simulink library "AeroLib"  (Simulink 6.0)
settings: Solver=ode45  SolverMode=SingleTasking  StartTime=0.0  StopTime=10.0  RelTol=1e-3
undefined symbols (not defined in the file): Aero, Ap, Atm, Control, Controls, Eng, Flight_cg, Flight_DamperON, Flight_delta_isa, Flight_DeltaSpiral, Flight_InertiaSelect, Flight_ixx, Flight_ixz, Flight_iyy, Flight_izz, Flight_latitude, Flight_LoiterLenght, Flight_LoiterMode, Flight_LoiterRadius, Flight_longitude, Flight_MaxTargetPoints, Flight_SensorsON, Flight_TimeStep, Flight_TowerWind_X, Flight_TowerWind_Y, Flight_TowerWind_Z, Flight_TowerWindON, Flight_Trimming, Flight_TurbON, Flight_weight, Flight_WindGustON, Flight_WindShearON, Flight_ycg, Flight_zcg, Geom, Lgear, Mass, PEG_CDwbnp, PEG_CLht, PEG_CLht_elev, PEG_CLwbnp, PEG_CMht, PEG_CMwbnp, PEG_CNbeta, PEG_CNr, PEG_CNrud, PEG_CRail, PEG_CRbeta, PEG_CRp, PEG_CRrud, PEG_CYbeta, PEG_CYrud, pow, Sensors
libraries: AeroLib x133, simulink3 x49, simulink x37, aerospace x11
(part 1 of 7)
settings Model: LastModifiedBy=MarcoP
settings OptimizationCC: BooleanDataType=off
settings DebuggingCC: SolverPrmCheckMsg=none
settings HardwareCC: TargetUnknown=on

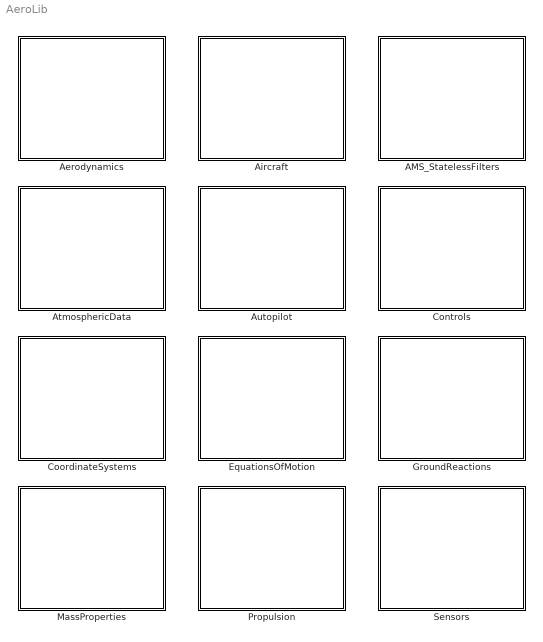
== system AeroLib ==
  AMS_StatelessFilters : Subsystem
      mask Display: image(imread('Filters.bmp','bmp'))
  Aerodynamics : Subsystem
      mask Display: image(imread('Aero.bmp','bmp'))
  Aircraft : Subsystem
      mask Type: Aircraft library
      mask Display: image(imread('Aircraft.bmp','bmp'))
  AtmosphericData : Subsystem
      mask Display: image(imread('Atm.bmp','bmp'))
  Autopilot : Subsystem
      mask Display: image(imread('Autopilot.bmp','bmp'))
  Controls : Subsystem
      mask Display: image(imread('Ctrl.bmp','bmp'))
  CoordinateSystems : Subsystem
      mask Display: image(imread('CoordSys.bmp','bmp'))
  EquationsOfMotion : Subsystem
      mask Display: image(imread('EQM.bmp','bmp'))
  GroundReactions : Subsystem
      mask Display: image(imread('Ground.bmp','bmp'))
  MassProperties : Subsystem
      mask Display: image(imread('Mass.bmp','bmp'))
  Propulsion : Subsystem
      mask Display: image(imread('Prop.bmp','bmp'))
  Sensors : Subsystem
      mask Display: image(imread('Sensors.bmp','bmp'))

== system AeroLib/AMS_StatelessFilters ==
  note: NB: The high pass has a
      | gain error of tau at high frequencies
  FlightTrim_Switch : Subsystem
      mask Help: See AeroLib Reference Manual.
      mask Display: patch([0 0.45 0.45 0.55 0.55 1], [0 0 1 1 0 0], [0 0 0]);
  Stateless_Filter_Reset : Subsystem
      mask Help: See AeroLib Reference Manual.
      mask Display: patch([0 0.45 0.45 0.55 0.55 1], [0 0 1 1 0 0], [0 0 0]);
  Stateless_HighPass : Subsystem
      mask Help: See AeroLib Reference Manual.
      mask Display: patch([0 0.4 0.4 0.6 0.6 1], [0 0 1 1 0 0], [0 0 0]);
  Stateless_Integrator : Subsystem
      mask Help: See AeroLib Reference Manual.
      mask Display: patch([0 0.4 0.4 0.6 0.6 1], [0 0 1 1 0 0], [0 0 0]);
  Stateless_LeadLag : Subsystem
      mask Help: See AeroLib Reference Manual.
      mask Display: patch([0 0.4 0.4 0.6 0.6 1], [0 0 1 1 0 0], [0 0 0]);
  Stateless_LimIntegrator : Subsystem
      mask Help: See AeroLib Reference Manual.
      mask Display: patch([0 0.4 0.4 0.6 0.6 1], [0 0 1 1 0 0], [0 0 0]);
  Stateless_LowPass : Subsystem
      mask Help: See AeroLib Reference Manual.
      mask Display: patch([0 0.4 0.4 0.6 0.6 1], [0 0 1 1 0 0], [0 0 0]);
  Stateless_RateLimiter : Subsystem
      mask Help: See AeroLib Reference Manual.
      mask Display: patch([0 0.4 0.4 0.6 0.6 1], [0 0 1 1 0 0], [0 0 0]);

== system AeroLib/Aerodynamics ==
  Aero NonDim_Rates : Subsystem  mask{Bref=Geom.Wing.bref, Cref=Geom.Wing.cref}
      mask prompts: Bref "Wing Span"; Cref "Wing MAC"
  Aerodynamic_Linear_Static : Subsystem
  Aerodynamics_Generic : Subsystem
      mask Help: See AeroLib Reference Manual.
      mask Display: patch( [0 0.4 0.4 0.6 0.6 1], [0 0 1 1 0 0],  [1 0 0])
  Aerodynamics_Pioneer : Subsystem
      mask Help: See AeroLib Reference Manual.
      mask Display: patch( [0 0.4 0.4 0.6 0.6 1], [0 0 1 1 0 0],  [1 0 0])
  INIT_Arms : Subsystem  mask{zacnp=Geom.Nacelle.zacnp, xacnp=Geom.Nacelle.xacnp, zacvt=Geom.Vtail.zacvt, xacvt=Geom.Vtail.xacvt, zacht=Geom.Htail.zacht, yacht=Geom.Htail.yacht, xacht=Geom.Htail.xacht, Cref=Geom.Wing.cref, Bref=Geom.Wing.bref}
      mask prompts: zacnp "(znp - zac)/span"; xacnp "(xnp - xac)/span"; zacvt "(zacvt -zac)/span"; xacvt "(xacvt - xac)/span"; zacht "(zacht -zac)/mac"; yacht "(yacht -yac)/span"; xacht "(xacht - xac)/mac"; Cref "Wing MAC"; Bref "Wing Span"
      mask help:
      | Htail - Horizontal Tail
      | Vtail - Vertical Tail
      | np - nacelle pilon
  Loads : Subsystem  mask{Bref=Geom.Wing.bref, Cref=Geom.Wing.cref, Sw=Geom.Wing.sw}
      mask prompts: Bref "Wing Span"; Cref "Wing MAC"; Sw "Wing Area"
  Transf to CG : Subsystem  mask{Bref=Geom.Wing.bref, Cref=Geom.Wing.cref}
      mask prompts: Bref "Wing Span"; Cref "Wing MAC"

== system AeroLib/Aircraft ==
  Generic_Aircraft : Subsystem
      mask Help: See AeroLib Reference Manual.
      mask Display:
      | patch( [0 0.07 0.19 0.09 0.02 0.07 0], [1 0.6 0.6 0.75 0.75 0.6 1], [0 0.7 1])
      | patch( [0 0.09 0.21 0.07 0], [0.52 0.52 0.6 0.6 0.52], [0 0.7 1])
      | patch( [0 0.25 0.37 0.59 0.4 0.25 0], [0 0.32 0.32 0.5 0.5 0.32 0], [0 0.7 1])
      | patch( [0.21 0.86 0.86 0.07 0.21], [0.5 0.5 0.6 0.6 0.5], [0 0.7 1])
      | patch( [0.86 1 1 0.86 0.86], [0.5 0.5 0.52 0.6 0.5], [0 0.7 1])
      | patch( [0.48 0.67 0.75 0.65 0.48], [0.6 0.6 0.7 0.7 0.6], [0 0.7 1])
  Pioneer_Aircraft : Subsystem
      mask Help: See AeroLib Reference Manual.
      mask Display:
      | patch( [0 0.07 0.19 0.09 0.02 0.07 0], [1 0.6 0.6 0.75 0.75 0.6 1], [0 0.7 1])
      | patch( [0 0.09 0.21 0.07 0], [0.52 0.52 0.6 0.6 0.52], [0 0.7 1])
      | patch( [0 0.25 0.37 0.59 0.4 0.25 0], [0 0.32 0.32 0.5 0.5 0.32 0], [0 0.7 1])
      | patch( [0.21 0.86 0.86 0.07 0.21], [0.5 0.5 0.6 0.6 0.5], [0 0.7 1])
      | patch( [0.86 1 1 0.86 0.86], [0.5 0.5 0.52 0.6 0.5], [0 0.7 1])
      | patch( [0.48 0.67 0.75 0.65 0.48], [0.6 0.6 0.7 0.7 0.6], [0 0.7 1])

== system AeroLib/AtmosphericData ==
  Atmosphere : Subsystem  mask{ISA=Flight_delta_isa, g=9.806, gamma=1.4, R=287.0529, L=0.0065, h_trop=11000, P0=101325.0, T0=288.15}
      mask prompts: ISA "Delta_ISA_C"; g "Gravity Acceleration [m/s2]"; gamma "Ratio of Specific Heats"; R "Characteristic Gas Constant [J/Kg/K]"; L "Lapse Rate [K/m]"; h_trop "Height of Troposphere [m]"; P0 "Pressure at sea level [N/m2]"; T0 "Ambient Temperature at Sea Level [K]"
      mask Display: patch([0 0.45 0.45 0.55 0.55 1], [0 0 1 1 0 0], [0 0.9 0.2])
  AtmosphericData_FAA_gust : Subsystem
      settings: RTWSystemCode=Function  RTWFcnNameOpts=Use subsystem name  RTWFileNameOpts=Use subsystem name
      mask Help: See AeroLib Reference Manual.
      mask Display: patch( [0 0.4 0.4 0.6 0.6 1], [0 0 1 1 0 0],  [0 0.9 0.2])
  FAA_Std_Gust : Subsystem
      mask Help: See AeroLib Reference Manual.
      mask Display: patch(  [0 0.45 0.45 0.55 0.55 1], [0 0 1 1 0 0],  [0 0.9 0.2])
  Simple_Wind_Gust : Subsystem  mask{WGfac=3, F=2.5, Wgain=-0.05}
      mask Help: See AeroLib Reference Manual.
      mask Display: patch(  [0 0.45 0.45 0.55 0.55 1], [0 0 1 1 0 0],  [0 0.9 0.2])

== system AeroLib/Autopilot ==
  AutoPilot_Out : Subsystem
      mask Display: disp('Empty')
  Autopilot : Subsystem
      settings: RTWSystemCode=Function  RTWFcnNameOpts=Use subsystem name  RTWFileNameOpts=Use subsystem name
      mask Help: See AeroLib Reference Manual.
      mask Display: patch( [0 0.4 0.4 0.6 0.6 1], [0 0 1 1 0 0],  [0 0.7 1])
  Counter_Point : Subsystem  mask{MinDist=Ap.Target.MinDist}
      mask prompts: MinDist "Minimal Distance"
  GeodCoor to XY : Subsystem
  Geod_Target_Errors : Subsystem
  PID : Subsystem  mask(PID(2) Controller){P=Ap.Alt.pgain, I=Ap.Alt.igain, D=0, Lim_I=Ap.Alt.igainLim, Lim_Err=Ap.Alt.LimAlt, Lim_Com=50}
      mask prompts: P "Proportional:"; I "Integral:"; D "Derivative:"; Lim_I "Limit Integral"; Lim_Err "Limit Error"; Lim_Com "Limit Comand"
      mask help:
      | Enter Proportional(P), Integral(I), and Derivative(D) terms.
      | P+I/s+Ds
      mask Help: This block implements a PID controller where parameters are entered for the Proportional, Integral and Derivative and divisor terms. Unmask this block to see how it works. The derivative term is implemented using an s/(s/N +1)  transfer function block. Making N large can create a "stiff" system.
      mask Display: disp('PID')
  Target_Errors : Subsystem

== system AeroLib/Controls ==
  Simple_Aileron_Actuator : Subsystem  mask{tau=Controls.Ail.Gain, ratio=Control.Wheel.Ratio, up=Controls.Ail.MaxAngle, low=-Controls.Ail.MaxAngle}
      mask prompts: tau "Time constant"; ratio "Aileron ratio"; up "Up limit"; low "Low limit"
      mask Help: See AeroLib Reference Manual.
      mask Display: patch( [0 0.5 0.5 0 0 0.5 0.5 1 0 0], [0 0 0.2 0.2 0.8 0.8 1 1 1 0],  [1 1 0.6])
  Simple_Controls : Subsystem
      mask Help: See AeroLib Reference Manual.
      mask Display: patch( [0 0.4 0.4 0.6 0.6 1], [0 0 1 1 0 0], [1 0 0.8])
  Simple_Elevator_Actuator : Subsystem  mask{tau=Controls.Elev.Gain, up=Controls.Elev.MaxPos, low=Controls.Elev.MaxNeg}
      mask prompts: tau "Time constant"; up "Up limit"; low "Low limit"
      mask Help: See AeroLib Reference Manual.
      mask Display: patch( [0 0.5 0.5 0 0 0.5 0.5 1 0 0], [0 0 0.2 0.2 0.8 0.8 1 1 1 0],  [1 1 0.6])
  Simple_Flap_Actuator : Subsystem  mask{flap_pos=Controls.flapslat, flap_defl=Controls.flap.Defl, flap_rate=Controls.flap.Rate}
      mask prompts: flap_pos "Flap Position"; flap_defl "Flap Deflection"; flap_rate "Flap Rate Limit"
      mask Help: See AeroLib Reference Manual.
      mask Display: patch( [0 0.5 0.5 0 0 0.5 0.5 1 0 0], [0 0 0.1 0.1 0.9 0.9 1 1 1 0],  [1 1 0.6])
  Simple_Rudder_Actuator : Subsystem  mask{tau=Controls.Rudder.Gain, up=Controls.Rudder.MaxAngle, low=-Controls.Rudder.MaxAngle}
      mask prompts: tau "Time constant"; up "Up limit"; low "Low limit"
      mask Help: See AeroLib Reference Manual.
      mask Display: patch( [0 0.5 0.5 0 0 0.5 0.5 1 0 0], [0 0 0.2 0.2 0.8 0.8 1 1 1 0],  [1 1 0.6])
  Simple_Stab_Actuator : Subsystem  mask{gain=Controls.Stab.Gain, up=Controls.Stab.MaxPos, low=Controls.Stab.MaxNeg}
      mask prompts: up "Up Limit"; low "Low Limit"
      mask Help: See AeroLib Reference Manual.
      mask Display: patch( [0 0.5 0.5 0 0 0.5 0.5 1 0 0], [0 0 0.2 0.2 0.8 0.8 1 1 1 0],  [1 1 0.6])

== system AeroLib/CoordinateSystems ==
  BOA2LEF : Subsystem
      settings: RTWSystemCode=Function  RTWFcnNameOpts=Use subsystem name  RTWFileNameOpts=Use subsystem name
      mask Help: See AeroLib Reference Manual.
      mask Display: patch( [0 0.5 0.5 1 1 0.5 0.5 1 1 0.5], [0 0 1 1 0.6 0.6 0.4 0.4 0 0], [1 1 0.6])
  EUL2DCM : Subsystem
      settings: RTWSystemCode=Function  RTWFcnNameOpts=Use subsystem name  RTWFileNameOpts=Use subsystem name
      mask Help: See AeroLib Reference Manual.
      mask Display: patch( [0 0.5 0.5 0 0 0.5 0.5 1 0 0], [0 0 0.4 0.4 0.6 0.6 1 1 1 0], [1 0 0])
  EUL2QUA : Subsystem
      settings: RTWSystemCode=Function  RTWFcnNameOpts=Use subsystem name  RTWFileNameOpts=Use subsystem name
      mask Help: See AeroLib Reference Manual.
      mask Display: patch( [0 0.5 0.5 0 0 0.5 0.5 1 0 0], [0 0 0.4 0.4 0.6 0.6 1 1 1 0], [0 0 .9])
  QUA2DCM : Subsystem
      settings: RTWSystemCode=Function  RTWFcnNameOpts=Use subsystem name  RTWFileNameOpts=Use subsystem name
      mask Help: See AeroLib Reference Manual.
      mask Display: patch( [0 0.5 0.5 1 1 0.5 0.5 1 1 0.5], [0 0 1 1 0.6 0.6 0.4 0.4 0 0], [1 0 0])
  QUA2EUL : Subsystem
      settings: RTWSystemCode=Function  RTWFcnNameOpts=Use subsystem name  RTWFileNameOpts=Use subsystem name
      mask Help: See AeroLib Reference Manual.
      mask Display: patch( [0 0.5 0.5 1 1 0.5 0.5 1 1 0.5], [0 0 1 1 0.6 0.6 0.4 0.4 0 0], [0 0 .9])
  STA2BOA : Subsystem
      settings: RTWSystemCode=Function  RTWFcnNameOpts=Use subsystem name  RTWFileNameOpts=Use subsystem name
      mask Help: See AeroLib Reference Manual.
      mask Display: patch( [0 0.5 0.5 1 1 0.5 0.5 1 1 0.5], [0 0 1 1 0.6 0.6 0.4 0.4 0 0], [1 1 0.6])
  WND2STA : Subsystem
      settings: RTWSystemCode=Function  RTWFcnNameOpts=Use subsystem name  RTWFileNameOpts=Use subsystem name
      mask Help: See AeroLib Reference Manual.
      mask Display: patch( [0 0.5 0.5 1 1 0.5 0.5 1 1 0.5], [0 0 1 1 0.6 0.6 0.4 0.4 0 0], [1 1 0.6])

== system AeroLib/EquationsOfMotion ==
  Equations_of_Motion : Subsystem
      mask Type: SampleMaskedBlock
      mask Help: See AeroLib Reference Manual.
      mask Display: patch( [0 0.5 0.5 1 1 0.5 0.5 1 1 0.5], [0 0 1 1 0.6 0.6 0.4 0.4 0 0], [0 0 1])
  External_Forces_and_Moments : Subsystem
      mask Help: See AeroLib Reference Manual.
      mask Display: patch( [0 0.5 0.5 1 1 0.5 0.5 1 1 0.5], [0 0 1 1 0.92 0.92 0.08 0.08 0 0], [0 0 1])

== system AeroLib/GroundReactions ==
  Gear_Out : Subsystem
      mask Display: disp('Empty')
  Landing_Gear : Subsystem
      settings: RTWSystemCode=Function  RTWFcnNameOpts=Use subsystem name  RTWFileNameOpts=Use subsystem name
      mask Help: See AeroLib Reference Manual.
      mask Display: patch( [0 0.4 0.4 0.6 0.6 1], [0 0 1 1 0 0],  [.8 0.8 .8])

== system AeroLib/MassProperties ==
  Mass_Properties : Subsystem
      settings: RTWSystemCode=Function  RTWFcnNameOpts=Use subsystem name  RTWFileNameOpts=Use subsystem name
      mask Help: See AeroLib Reference Manual.
      mask Display: patch( [0 0.4 0.4 0.6 0.6 1], [0 0 1 1 0 0],  [0 0 0])

== system AeroLib/Propulsion ==
  Booster : Subsystem  mask{Booster_Time=Eng.Booster.Time, Xpos=Geom.Eng.Booster.Xpos, Ypos=Geom.Eng.Booster.Ypos, Zpos=Geom.Eng.Booster.Zpos, Booster_Thrust=Eng.Booster.Thrust, pitch=Geom.Eng.Booster.pitch}
      mask prompts: Booster_Time "Booster_Time [sec]"; Xpos "Booster_Xpos"; Ypos "Booster_Ypos"; Zpos "Booster_Zpos"; Booster_Thrust "Average_Thrust"; pitch "Booster_Pitch [Deg]"
      mask Help: See AeroLib Reference Manual.
  Engine_Empty : Subsystem  mask{Xthrust=10000}
      mask prompts: Xthrust "Xthrust [N]"
  Engine_Transient : Subsystem
      mask Help: See AeroLib Reference Manual.
  Fixed_Pitch_Propeller : Subsystem  mask{reduc=Eng.Prop.reduc, prop_diam=Eng.Prop.diam}
      mask prompts: reduc "Reduction"; prop_diam "Propeller Diameter"
      mask Help: See AeroLib Reference Manual.
  Jet_Engine : Subsystem
      mask Help: See AeroLib Reference Manual.
  Piston_Engine : Subsystem
      mask Help: See AeroLib Reference Manual.
  Piston_Engine_Propeller : Subsystem
      mask Help: See AeroLib Reference Manual.
  Piston_Engine_Propeller_system : Subsystem
      mask Help: See AeroLib Reference Manual.
      mask Display: patch( [0 0.4 0.4 0.6 0.6 1], [0 0 1 1 0 0],  [1 0.5 0])
  Propeller_Power_Demand : Subsystem  mask{D=Eng.Prop.diam}
      mask prompts: D "Propeller Diameter [m]"
      mask Help: See AeroLib Reference Manual.
  Thrust_Components : Subsystem  mask{grav=Atm.grav, Sw=Geom.Wing.sw, Xpos=Geom.Eng.Xpos, Ypos=Geom.Eng.Ypos, Zpos=Geom.Eng.Zpos, pitch=Geom.Eng.pitch, toeout=Geom.Eng.toeout}
      mask prompts: grav "Atm Gravity"; Sw "Wing Area"; Xpos "Engine_Xpos"; Ypos "Engine_Ypos"; Zpos "Engine_Zpos"; pitch "Engine_pitch [rad]"; toeout "Engine_toeout [rad]"
      mask Help: See AeroLib Reference Manual.
  Twin_Jet_Engine_system : Subsystem
      mask Help: See AeroLib Reference Manual.
      mask Display: patch( [0 0.4 0.4 0.6 0.6 1], [0 0 1 1 0 0], [1 0.5 0])
  Variable_Pitch_Propeller : Subsystem  mask{reduc=, prop_diam=}
      mask prompts: reduc "Reduction"; prop_diam "Propeller Diameter"
      mask Help: See AeroLib Reference Manual.

== system AeroLib/Sensors ==
  Air_Data_Computer : Subsystem
      mask Help: See AeroLib Reference Manual.
      mask Display: patch( [0 0.5 0.5 1 1 0.5 0.5 1 1 0.5], [0 0 1 1 0.8 0.8 0.2 0.2 0 0], [0 0.6 0])
  Flight_System_Computer : Subsystem  mask{Kgps=Sensors.FSC.Kgps, Kins=Sensors.FSC.Kins}
      mask prompts: Kgps "GPS weight coefficient"; Kins "INS weight coefficient"
      mask Help: See AeroLib Reference Manual.
      mask Display: patch( [0 0.5 0.5 1 1 0.5 0.5 1 1 0.5], [0 0 1 1 0.8 0.8 0.2 0.2 0 0], [0 0.6 0])
  Gauss_Markov : Subsystem  mask{Seed=, tau=, Var=}
      mask prompts: tau "Correlation time"; Var "Variance"
      mask Help: See AeroLib Reference Manual.
  Global_Positioning_System : Subsystem  mask(GPS Position-Velocity){Time_delay=Sensors.GPS.TimeDelay, Var=Sensors.GPS.Var, Seed=Sensors.GPS.Seed, Time=Sensors.GPS.CorTime}
      mask prompts: Time_delay "Time Delay"; Var "Variance"; Time "Correlation time"
      mask Help: See AeroLib Reference Manual.
      mask Display: patch( [0 0.5 0.5 1 1 0.5 0.5 1 1 0.5], [0 0 1 1 0.8 0.8 0.2 0.2 0 0], [0 0.6 0])
  Inertial_Reference_Unit : Subsystem  mask{PlatformDev=Sensors.IRU.PlatDev, MagDev=Sensors.IRU.MagDev}
      mask prompts: PlatformDev "Patform Heading Deviation (deg)"; MagDev "Magnetic Heading Deviation (deg)"
      mask Help: See AeroLib Reference Manual.
      mask Display: patch( [0 0.5 0.5 1 1 0.5 0.5 1 1 0.5], [0 0 1 1 0.8 0.8 0.2 0.2 0 0], [0 0.6 0])
  Navigation_Sensors : Subsystem
      settings: RTWSystemCode=Function  RTWFcnNameOpts=Use subsystem name  RTWFileNameOpts=Use subsystem name
      mask Help: See AeroLib Reference Manual.
      mask Display: patch( [0 0.4 0.4 0.6 0.6 1], [0 0 1 1 0 0],  [0 0.6 0])
  Random Walk : Subsystem  mask{Seed=, Var=}
      mask prompts: Var "Variance"
      mask Help: See AeroLib Reference Manual.
  Simple_Sensor : Subsystem  mask{Var=Sensors.ADC.Var, Seed=Sensors.ADC.Seed, Max=60000, Min=-300, Time_Const=Sensors.ADC.TimeConst}
      mask prompts: Var "Variance"; Max "Upper limit"; Min "Lower limit"; Time_Const "Time Constant"
      mask Help: See AeroLib Reference Manual.

== system AeroLib/AMS_StatelessFilters/FlightTrim_Switch ==
  In1 : Inport  Port=1  LatchInput=off
  Constant1 : Constant  Value=Flight_Trimming
  DeadZone : DeadZone  LowerValue=-eps  UpperValue=eps  SaturateOnIntegerOverflow=on
  Switch : Switch  Threshold=0.5  SaturateOnIntegerOverflow=on  InputSameDT=on
  Out1 : Outport
  wires:
  DeadZone/1 -> Switch/3
  Constant1/1 -> Switch/2
  In1/1 -> DeadZone/1, Switch/1
  Switch/1 -> Out1/1

== system AeroLib/AMS_StatelessFilters/Stateless_Filter_Reset ==
  Bus Creator : BusCreator  DialogController=Simulink.DDGSource_Bus  Inputs=2
  Clock : Clock
      settings: Decimation=10
  Fcn : Fcn  Expr=u <= 0 || Flight_Trimming>0.5
  LastTime : Memory
  Sum1 : Sum  Inputs=|+-  SaturateOnIntegerOverflow=on  InputSameDT=on
  Reset_Out : Outport
  wires:
  Bus Creator/1 -> Reset_Out/1
  LastTime/1 -> Sum1/2
  Sum1/1 -> Bus Creator/2  "TimeStep"
  Fcn/1 -> Bus Creator/1  "Filter_Reset"
  Clock/1 -> LastTime/1, Sum1/1, Fcn/1

== system AeroLib/AMS_StatelessFilters/Stateless_HighPass ==
  Reset : Inport  Port=1  LatchInput=off
  X : Inport  Port=2  LatchInput=off
  Tau : Inport  Port=3  LatchInput=off
  Bus Selector : BusSelector  DialogController=Simulink.DDGSource_Bus  OutputSignals=Filter_Reset,TimeStep
  Filter : Memory
  Freq : Product  Inputs=*/*  SaturateOnIntegerOverflow=on  InputSameDT=on
  Sum1 : Sum  Inputs=|+-  SaturateOnIntegerOverflow=on  InputSameDT=on
  Sum3 : Sum  Inputs=|++  SaturateOnIntegerOverflow=on  InputSameDT=on
  Sum4 : Sum  Inputs=|-+  SaturateOnIntegerOverflow=on  InputSameDT=on
  Sw : Switch  Threshold=0.5  SaturateOnIntegerOverflow=on  InputSameDT=on
  Sw1 : Switch  Threshold=0.5  SaturateOnIntegerOverflow=on  InputSameDT=on
  X0 : Constant  Value=0
  XLead : Outport
  wires:
  Reset/1 -> Bus Selector/1
  X/1 -> Sum4/2, Sw/1, Sum1/1
  Filter/1 -> Sum3/2, Sum1/2, Sum4/1  "LastX"
  Sum1/1 -> Freq/3
  Tau/1 -> Freq/2
  Bus Selector/2 -> Freq/1
  Sw/1 -> Filter/1  "LastX"
  Bus Selector/1 -> Sw1/2, Sw/2
  Sum3/1 -> Sw/3
  Freq/1 -> Sum3/1
  Sum4/1 -> Sw1/3
  Sw1/1 -> XLead/1
  X0/1 -> Sw1/1

== system AeroLib/AMS_StatelessFilters/Stateless_Integrator ==
  Reset : Inport  Port=1  LatchInput=off
  X0 : Inport  Port=2  LatchInput=off
  Xdot : Inport  Port=3  LatchInput=off
  Bus Selector : BusSelector  DialogController=Simulink.DDGSource_Bus  OutputSignals=Filter_Reset,TimeStep
  Filter : Memory
  Freq : Product  SaturateOnIntegerOverflow=on  InputSameDT=on
  Sum3 : Sum  Inputs=|++  SaturateOnIntegerOverflow=on  InputSameDT=on
  Sw : Switch  Threshold=0.5  SaturateOnIntegerOverflow=on  InputSameDT=on
  Sw1 : Switch  Threshold=0.5  SaturateOnIntegerOverflow=on  InputSameDT=on
  X : Outport
  wires:
  Reset/1 -> Bus Selector/1
  Sw/1 -> Filter/1
  Bus Selector/1 -> Sw/2, Sw1/2  "<Filter_Reset>"
  Bus Selector/2 -> Freq/1  "<TimeStep>"
  Sum3/1 -> Sw/3
  X0/1 -> Sw/1, Sw1/1
  Xdot/1 -> Freq/2
  Freq/1 -> Sum3/1  "XdotDT"
  Filter/1 -> Sum3/2, Sw1/3  "LastX"
  Sw1/1 -> X/1

== system AeroLib/AMS_StatelessFilters/Stateless_LeadLag ==
  Reset : Inport  Port=1  LatchInput=off
  X0 : Inport  Port=2  LatchInput=off
  X : Inport  Port=3  LatchInput=off
  Tau_num : Inport  Port=4  LatchInput=off
  Tau_den : Inport  Port=5  LatchInput=off
  Product : Product  Inputs=**/  SaturateOnIntegerOverflow=on  InputSameDT=on
  Stateless_LowPass : AeroLib/AMS_StatelessFilters/Stateless_LowPass
  Sum : Sum  Inputs=-+|  SaturateOnIntegerOverflow=on  InputSameDT=on
  Sum1 : Sum  Inputs=++|  SaturateOnIntegerOverflow=on  InputSameDT=on
  XLeadLag : Outport
  wires:
  Sum1/1 -> XLeadLag/1
  Product/1 -> Sum1/2
  Sum/1 -> Product/1
  Tau_den/1 -> Stateless_LowPass/4, Product/3
  Tau_num/1 -> Product/2
  X/1 -> Stateless_LowPass/3, Sum/2
  Reset/1 -> Stateless_LowPass/1
  X0/1 -> Stateless_LowPass/2
  Stateless_LowPass/1 -> Sum1/1, Sum/1

== system AeroLib/AMS_StatelessFilters/Stateless_LimIntegrator ==
  Reset : Inport  Port=1  LatchInput=off
  X0 : Inport  Port=2  LatchInput=off
  Xdot : Inport  Port=3  LatchInput=off
  Xmin : Inport  Port=4  LatchInput=off
  Xmax : Inport  Port=5  LatchInput=off
  Bus Selector : BusSelector  DialogController=Simulink.DDGSource_Bus  OutputSignals=Filter_Reset,TimeStep
  Filter1 : Memory
  Freq1 : Product  SaturateOnIntegerOverflow=on  InputSameDT=on
  MinMax3 : MinMax  Function=max  Inputs=2  SaturateOnIntegerOverflow=on  InputSameDT=on
  MinMax4 : MinMax  Inputs=2  SaturateOnIntegerOverflow=on  InputSameDT=on
  Sum1 : Sum  Inputs=|++  SaturateOnIntegerOverflow=on  InputSameDT=on
  Sw1 : Switch  Threshold=0.5  SaturateOnIntegerOverflow=on  InputSameDT=on
  Sw2 : Switch  Threshold=0.5  SaturateOnIntegerOverflow=on  InputSameDT=on
  X : Outport
  wires:
  Bus Selector/1 -> Sw2/2, Sw1/2  "<Filter_Reset>"
  Bus Selector/2 -> Freq1/1  "<TimeStep>"
  Reset/1 -> Bus Selector/1
  Xmin/1 -> MinMax3/2
  Xmax/1 -> MinMax4/2
  Sum1/1 -> Sw1/3
  X0/1 -> Sw1/1, Sw2/1
  Xdot/1 -> Freq1/2
  Freq1/1 -> Sum1/1  "XdotDT"
  Filter1/1 -> Sum1/2, Sw2/3  "LastX"
  Sw2/1 -> X/1
  Sw1/1 -> MinMax3/1
  MinMax3/1 -> MinMax4/1
  MinMax4/1 -> Filter1/1

== system AeroLib/AMS_StatelessFilters/Stateless_LowPass ==
  Reset : Inport  Port=1  LatchInput=off
  X0 : Inport  Port=2  LatchInput=off
  X : Inport  Port=3  LatchInput=off
  Tau : Inport  Port=4  LatchInput=off
  Bus Selector : BusSelector  DialogController=Simulink.DDGSource_Bus  OutputSignals=Filter_Reset,TimeStep
  Filter : Memory
  Freq : Product  Inputs=*/*  SaturateOnIntegerOverflow=on  InputSameDT=on
  Sum1 : Sum  Inputs=|+-  SaturateOnIntegerOverflow=on  InputSameDT=on
  Sum3 : Sum  Inputs=|++  SaturateOnIntegerOverflow=on  InputSameDT=on
  Sw : Switch  Threshold=0.5  SaturateOnIntegerOverflow=on  InputSameDT=on
  Sw1 : Switch  Threshold=0.5  SaturateOnIntegerOverflow=on  InputSameDT=on
  XLag : Outport
  wires:
  Bus Selector/1 -> Sw1/2, Sw/2  "<Filter_Reset>"
  Reset/1 -> Bus Selector/1
  Sw1/1 -> XLag/1
  Filter/1 -> Sw1/3, Sum3/2, Sum1/2  "LastX"
  Sum1/1 -> Freq/3
  Tau/1 -> Freq/2
  Bus Selector/2 -> Freq/1  "<TimeStep>"
  Sw/1 -> Filter/1  "LastX"
  Sum3/1 -> Sw/3
  X0/1 -> Sw/1, Sw1/1
  X/1 -> Sum1/1
  Freq/1 -> Sum3/1

== system AeroLib/AMS_StatelessFilters/Stateless_RateLimiter ==
  Reset : Inport  Port=1  LatchInput=off
  X : Inport  Port=2  SampleTime=[0.01,0]  LatchInput=off
  Xdotmin : Inport  Port=3  SampleTime=[0.01,0]  LatchInput=off
  Xdotmax : Inport  Port=4  SampleTime=[0.01,0]  LatchInput=off
  Bus Selector : BusSelector  DialogController=Simulink.DDGSource_Bus  OutputSignals=Filter_Reset,TimeStep
  LastTime : Memory  Orientation=left
  MinMax : MinMax  Inputs=2  SaturateOnIntegerOverflow=on  InputSameDT=on
  MinMax1 : MinMax  Function=max  Inputs=2  SaturateOnIntegerOverflow=on  InputSameDT=on
  Product : Product  SaturateOnIntegerOverflow=on  InputSameDT=on
  Product1 : Product  SaturateOnIntegerOverflow=on  InputSameDT=on
  Sum1 : Sum  Inputs=|++  SaturateOnIntegerOverflow=on  InputSameDT=on
  Sum2 : Sum  Inputs=++|  SaturateOnIntegerOverflow=on  InputSameDT=on
  Switch : Switch  Threshold=0.5  SaturateOnIntegerOverflow=on  InputSameDT=on
  Xr : Outport
  wires:
  Reset/1 -> Bus Selector/1
  MinMax1/1 -> Switch/3
  Sum1/1 -> MinMax1/1
  MinMax/1 -> MinMax1/2
  X/1 -> Switch/1, MinMax/1
  Sum2/1 -> MinMax/2
  Switch/1 -> Xr/1, LastTime/1
  Bus Selector/1 -> Switch/2
  Product1/1 -> Sum2/2
  LastTime/1 -> Sum2/1, Sum1/2
  Product/1 -> Sum1/1
  Xdotmax/1 -> Product1/2
  Xdotmin/1 -> Product/2
  Bus Selector/2 -> Product1/1, Product/1

== system AeroLib/Aerodynamics/Aero NonDim_Rates ==
  RatesRad : Inport  Port=1  LatchInput=off
  AlphaDot : Inport  Port=2  LatchInput=off
  TAS : Inport  Port=3  LatchInput=off
  Fcn : Fcn  Expr=u(1)*Cref/2/u(2)
  Fcn1 : Fcn  Expr=u(1)*Bref/2/u(4)
  Fcn2 : Fcn  Expr=u(3)*Bref/2/u(4)
  Fcn3 : Fcn  Expr=u(2)*Cref/2/u(4)
  Reshape : simulink3/Signals & Systems/Reshape  OutputDimensionality=1-D array  OutputDimensions=[1,1]
  non_dim rates (8) Mux_2 : Mux  Inputs=2
  non_dim rates (8) Mux_3 : Mux  Inputs=2
  Phat : Outport
  Rhat : Outport  Port=2
  Adothat : Outport  Port=3
  Qhat : Outport  Port=4
  wires:
  non_dim rates (8) Mux_3/1 -> Fcn/1
  non_dim rates (8) Mux_2/1 -> Fcn1/1, Fcn2/1, Fcn3/1
  TAS/1 -> non_dim rates (8) Mux_2/2, non_dim rates (8) Mux_3/2  "TAS"
  RatesRad/1 -> Reshape/1
  Fcn3/1 -> Qhat/1
  Fcn/1 -> Adothat/1
  Fcn2/1 -> Rhat/1
  Fcn1/1 -> Phat/1
  AlphaDot/1 -> non_dim rates (8) Mux_3/1
  Reshape/1 -> non_dim rates (8) Mux_2/1

== system AeroLib/Aerodynamics/Aerodynamic_Linear_Static ==
  From_Control : Inport  Port=1  LatchInput=off
  From_ATM : Inport  Port=2  LatchInput=off
  AeroCoefficients : Subsystem  mask{CLo=0.385, CL_Alpha=0.0834, CL_Elev=0.401*pi/180, CDo=0.06, CD_Alpha=0.43*pi/180, CY_Beta=-0.819*pi/180, CY_Rud=0.191*pi/180, CR_Beta=-0.23*pi/180, CR_Ail=-0.161*pi/180, CMo=0.194, CM_Alpha=-2.12*pi/180, CM_Elev=-1.76*pi/180, CN_Beta=0.109*pi/180, CN_Rud=-0.0917*pi/180}
  Bus Creator : BusCreator  DialogController=Simulink.DDGSource_Bus  Inputs=12
  Bus Selector : BusSelector  DialogController=Simulink.DDGSource_Bus  OutputSignals=Elev_deg,Rud_deg,Ail_deg
  Bus Selector1 : BusSelector  DialogController=Simulink.DDGSource_Bus  OutputSignals=DynPres_P,Beta,Alpha
  Constant4 : Constant  Value=Flight_cg
  Constant5 : Constant  Value=Flight_ycg
  Constant6 : Constant  Value=Flight_zcg
  Demux : Demux  Outputs=3
  INIT_Arms : AeroLib/Aerodynamics/INIT_Arms  zacnp=Geom.Nacelle.zacnp  xacnp=Geom.Nacelle.xacnp  zacvt=Geom.Vtail.zacvt  xacvt=Geom.Vtail.xacvt  zacht=Geom.Htail.zacht  yacht=Geom.Htail.yacht  xacht=Geom.Htail.xacht  Cref=Geom.Wing.cref  Bref=Geom.Wing.bref
  Loads : AeroLib/Aerodynamics/Loads  Bref=Geom.Wing.bref  Cref=Geom.Wing.cref  Sw=Geom.Wing.sw
  Mux : Mux  Inputs=3
  Stab2Body : AeroLib/Aerodynamics/Aerodynamics_Pioneer/Aero Total/Stab2Body  SimViewingDevice=off  DataTypeOverride=UseLocalSettings  MinMaxOverflowLogging=UseLocalSettings
      settings: Permissions=ReadWrite  RTWFcnNameOpts=Auto  RTWFileNameOpts=Auto
  Terminator : Terminator
  Terminator1 : Terminator
  Terminator2 : Terminator
  Transf to CG : AeroLib/Aerodynamics/Transf to CG  Bref=Geom.Wing.bref  Cref=Geom.Wing.cref
  Wind2Stab : AeroLib/Aerodynamics/Aerodynamics_Pioneer/Aero Total/Wind2Stab  SimViewingDevice=off  DataTypeOverride=UseLocalSettings  MinMaxOverflowLogging=UseLocalSettings
      settings: Permissions=ReadWrite  RTWFcnNameOpts=Auto  RTWFileNameOpts=Auto
  Aero_Out : Outport
  wires:
  From_ATM/1 -> Bus Selector1/1
  Bus Selector/3 -> AeroCoefficients/5(Aileron_deg)  "<Ail_deg>"
  Bus Selector/2 -> AeroCoefficients/4(Rudder_deg)  "<Rud_deg>"
  Bus Selector/1 -> AeroCoefficients/3(Elevator_deg)  "<Elev_deg>"
  From_Control/1 -> Bus Selector/1
  Bus Selector1/3 -> Stab2Body/1, AeroCoefficients/2(Alpha_deg)  "<Alpha>"
  Bus Selector1/2 -> Wind2Stab/1, AeroCoefficients/1(Beta_deg)  "<Beta>"
  Bus Selector1/1 -> Loads/1  "<DynPres_P>"
  INIT_Arms/4 -> Terminator/1
  Constant6/1 -> INIT_Arms/3
  Constant5/1 -> INIT_Arms/2
  Constant4/1 -> INIT_Arms/1
  INIT_Arms/1 -> Transf to CG/7
  INIT_Arms/2 -> Terminator1/1
  INIT_Arms/3 -> Terminator2/1
  AeroCoefficients/3(CL_Wind) -> Bus Creator/12, Mux/3  "CLw"
  AeroCoefficients/2(CY_Wind) -> Bus Creator/11, Mux/2  "CYw"
  Loads/6 -> Bus Creator/6  "Naero"
  Loads/5 -> Bus Creator/5  "Maero"
  Loads/1 -> Bus Creator/1  "Xaero"
  Loads/2 -> Bus Creator/2  "Yaero"
  Loads/3 -> Bus Creator/3  "Zaero"
  Loads/4 -> Bus Creator/4  "Laero"
  Bus Creator/1 -> Aero_Out/1
  AeroCoefficients/6(CN_body) -> Transf to CG/6
  AeroCoefficients/5(CM_body) -> Transf to CG/5
  AeroCoefficients/4(CR_body) -> Transf to CG/4
  Stab2Body/1 -> Demux/1
  Demux/3 -> Transf to CG/3
  Demux/2 -> Transf to CG/2
  Demux/1 -> Transf to CG/1
  Wind2Stab/1 -> Stab2Body/2
  Mux/1 -> Wind2Stab/2
  AeroCoefficients/1(CD_Wind) -> Bus Creator/10, Mux/1  "CDw"
  Transf to CG/6 -> Bus Creator/9, Loads/7  "CNcg"
  Transf to CG/5 -> Bus Creator/8, Loads/6  "CMcg"
  Transf to CG/4 -> Bus Creator/7, Loads/5  "CRcg"
  Transf to CG/3 -> Loads/4
  Transf to CG/2 -> Loads/3
  Transf to CG/1 -> Loads/2

== system AeroLib/Aerodynamics/Aerodynamics_Generic ==
  From_Ctrl : Inport  Port=1  LatchInput=off
  From_Atmos : Inport  Port=2  LatchInput=off
  From_EQM : Inport  Port=3  LatchInput=off
  From_Inputs : Inport  Port=4  LatchInput=off
  Aero_Loads : Subsystem
  Constant4 : Constant  Value=Flight_cg
  Constant5 : Constant  Value=Flight_ycg
  Constant6 : Constant  Value=Flight_zcg
  Drag : Subsystem
  INIT_Arms : AeroLib/Aerodynamics/INIT_Arms  zacnp=Geom.Nacelle.zacnp  xacnp=Geom.Nacelle.xacnp  zacvt=Geom.Vtail.zacvt  xacvt=Geom.Vtail.xacvt  zacht=Geom.Htail.zacht  yacht=Geom.Htail.yacht  xacht=Geom.Htail.xacht  Cref=Geom.Wing.cref  Bref=Geom.Wing.bref
  LIft : Subsystem
  Pitching Moment : Subsystem
  Rolling Moment : Subsystem
  Side Force : Subsystem
  Terminator : Terminator
  Terminator1 : Terminator
  Terminator2 : Terminator
  Yawing Moment : Subsystem
  Aero_Out : Outport
  wires:
  INIT_Arms/4 -> Terminator/1
  Constant6/1 -> INIT_Arms/3
  Constant5/1 -> INIT_Arms/2
  Constant4/1 -> INIT_Arms/1
  INIT_Arms/1 -> Aero_Loads/8(dcg2ac)
  INIT_Arms/2 -> Terminator1/1
  INIT_Arms/3 -> Terminator2/1
  Yawing Moment/1(YawM_Out) -> Aero_Loads/6(From_Yaw)
  Pitching Moment/1(PitchM_Out) -> Aero_Loads/5(From_Pitch)
  Rolling Moment/1(RollM_Out) -> Aero_Loads/4(From_Roll)
  LIft/1(Lift_Out) -> Aero_Loads/3(From_Lift), Pitching Moment/1(From_Lift)
  Drag/1(Drag_Out) -> Aero_Loads/1(From_Drag)
  Aero_Loads/1(Xaero) -> Aero_Out/1
  From_Ctrl/1 -> Drag/2(From_Ctrl), Rolling Moment/1(From_Ctrl), Pitching Moment/3(From_Ctrl), LIft/3(From_Ctrl), Yawing Moment/2(From_Ctrl), Side Force/1(From_Ctrl)
  From_Atmos/1 -> Drag/1(From_Atmos), Rolling Moment/2(From_Atmos), Aero_Loads/7(From_Atmos), Yawing Moment/3(From_Atmos), LIft/2(From_Atmos), Side Force/2(From_Atmos), Pitching Moment/2(From_Atmos)
  From_EQM/1 -> Side Force/3(From_EQM), LIft/1(From_EQM)
  From_Inputs/1 -> Drag/3(From_Inputs), Pitching Moment/4(From_Inputs)
  Side Force/1(SideF_Out) -> Aero_Loads/2(From_SideF), Rolling Moment/3(From_SideF), Yawing Moment/1(From_SideF)

== system AeroLib/Aerodynamics/Aerodynamics_Pioneer ==
  From_Ctrl : Inport  Port=1  LatchInput=off
  From_Atmos : Inport  Port=2  LatchInput=off
  From_EQM : Inport  Port=3  LatchInput=off
  Aero Total : Subsystem
  Aero_Coefficients : Subsystem
  Aero_Dynamic_Coefficients : Subsystem
  Bus Creator : BusCreator  DialogController=Simulink.DDGSource_Bus  Inputs=12
  Bus Selector1 : BusSelector  DialogController=Simulink.DDGSource_Bus  OutputSignals=Alpha,Beta,DynPres_P
  Constant4 : Constant  Value=Flight_cg
  Constant5 : Constant  Value=Flight_ycg
  Constant6 : Constant  Value=Flight_zcg
  Demux1 : Demux  Outputs=3
  INIT_Arms : AeroLib/Aerodynamics/INIT_Arms  zacnp=Geom.Nacelle.zacnp  xacnp=Geom.Nacelle.xacnp  zacvt=Geom.Vtail.zacvt  xacvt=Geom.Vtail.xacvt  zacht=Geom.Htail.zacht  yacht=Geom.Htail.yacht  xacht=Geom.Htail.xacht  Cref=Geom.Wing.cref  Bref=Geom.Wing.bref
  Terminator : Terminator
  Terminator1 : Terminator
  Terminator2 : Terminator
  Aero_Out : Outport
  wires:
  Aero_Coefficients/1(Moments_body) -> Aero Total/5(Moments_body)
  From_EQM/1 -> Aero_Dynamic_Coefficients/1(FromEqm)
  From_Atmos/1 -> Aero_Dynamic_Coefficients/2(FromAtm), Bus Selector1/1, Aero_Coefficients/2(From_ATM)
  From_Ctrl/1 -> Aero_Coefficients/1(From_Control)
  INIT_Arms/4 -> Terminator/1
  Constant6/1 -> INIT_Arms/3
  Constant5/1 -> INIT_Arms/2
  Constant4/1 -> INIT_Arms/1
  INIT_Arms/1 -> Aero Total/7(dcg2ac)
  INIT_Arms/2 -> Terminator1/1
  INIT_Arms/3 -> Terminator2/1
  Aero Total/6(Naero) -> Bus Creator/6  "Naero"
  Aero Total/5(Maero) -> Bus Creator/5  "Maero"
  Aero Total/1(Xaero) -> Bus Creator/1  "Xaero"
  Aero Total/2(Yaero) -> Bus Creator/2  "Yaero"
  Aero Total/3(Zaero) -> Bus Creator/3  "Zaero"
  Aero Total/4(Laero) -> Bus Creator/4  "Laero"
  Aero Total/8(CMcg) -> Bus Creator/8  "CMcg"
  Aero Total/9(CNcg) -> Bus Creator/9  "CNcg"
  Aero Total/7(CRcg) -> Bus Creator/7  "CRcg"
  Bus Creator/1 -> Aero_Out/1
  Aero_Dynamic_Coefficients/1(Cdyn) -> Aero Total/1(Cdyn)
  Aero_Coefficients/2(Forces_wind) -> Aero Total/6(Forces), Demux1/1
  Demux1/1 -> Bus Creator/10  "CDw"
  Demux1/2 -> Bus Creator/11  "CYw"
  Demux1/3 -> Bus Creator/12  "CLw"
  Bus Selector1/3 -> Aero Total/4(Qdyn_N)  "<DynPres_P>"
  Bus Selector1/2 -> Aero Total/3(Beta_deg)  "<Beta>"
  Bus Selector1/1 -> Aero Total/2(Alpha_deg)  "<Alpha>"

== system AeroLib/Aerodynamics/INIT_Arms ==
  cg : Inport  Port=1  LatchInput=off
  ycg : Inport  Port=2  LatchInput=off
  zcg : Inport  Port=3  LatchInput=off
  Gain : Gain  SaturateOnIntegerOverflow=on
  Mux : Mux  Inputs=3
  NP : Subsystem
  htail : Subsystem
  vtail : Subsystem
  xcg2ac : Fcn  Expr=(u-0.25)*Cref
  dcg2ac : Outport
  dhtac2cg : Outport  Port=2
  dvtac2cg : Outport  Port=3
  dnpac2cg : Outport  Port=4
  wires:
  Gain/1 -> dcg2ac/1
  NP/1(dnpac2cg) -> dnpac2cg/1
  cg/1 -> xcg2ac/1  "xcg"
  xcg2ac/1 -> htail/1(xcg2ac), vtail/1(xcg2ac), NP/1(xcg2ac), Mux/1
  ycg/1 -> Mux/2, htail/2(ycg2ac)
  zcg/1 -> Mux/3, NP/2(zcg2ac), vtail/2(zcg2ac), htail/3(zcg2ac)
  Mux/1 -> Gain/1
  htail/1(dhtac2cg) -> dhtac2cg/1
  vtail/1(dvtac2cg) -> dvtac2cg/1

== system AeroLib/Aerodynamics/Loads ==
  Qdyn : Inport  Port=1  LatchInput=off
  Cx : Inport  Port=2  LatchInput=off
  Cy : Inport  Port=3  LatchInput=off
  Cz : Inport  Port=4  LatchInput=off
  Cr : Inport  Port=5  LatchInput=off
  Cm : Inport  Port=6  LatchInput=off
  Cn : Inport  Port=7  LatchInput=off
  Product{1..6} (6 alike) : Product  SaturateOnIntegerOverflow=on  InputSameDT=on
  SW{1..6} (6 alike) : Gain  Gain=Sw  SaturateOnIntegerOverflow=on
  bref : Gain  Gain=Bref  SaturateOnIntegerOverflow=on
  bref1 : Gain  Gain=Bref  SaturateOnIntegerOverflow=on
  cref : Gain  Gain=Cref  SaturateOnIntegerOverflow=on
  Xaero : Outport
  Yaero : Outport  Port=2
  Zaero : Outport  Port=3
  Laero : Outport  Port=4
  Maero : Outport  Port=5
  Naero : Outport  Port=6
  wires:
  Product2/1 -> Yaero/1
  Product3/1 -> Zaero/1
  Product4/1 -> Laero/1
  Product5/1 -> Maero/1
  Product6/1 -> Naero/1
  Product1/1 -> Xaero/1
  Qdyn/1 -> Product5/2, Product6/2, Product4/2, Product3/2, Product2/2, Product1/2
  SW6/1 -> bref1/1
  SW5/1 -> cref/1
  SW4/1 -> bref/1
  SW3/1 -> Product3/1
  SW2/1 -> Product2/1
  SW1/1 -> Product1/1
  Cn/1 -> SW6/1
  Cm/1 -> SW5/1
  Cr/1 -> SW4/1
  Cz/1 -> SW3/1
  Cy/1 -> SW2/1
  Cx/1 -> SW1/1
  bref1/1 -> Product6/1
  cref/1 -> Product5/1
  bref/1 -> Product4/1

== system AeroLib/Aerodynamics/Transf to CG ==
  Cx : Inport  Port=1  LatchInput=off
  Cy : Inport  Port=2  LatchInput=off
  Cz : Inport  Port=3  LatchInput=off
  Cr_body : Inport  Port=4  LatchInput=off
  Cm_body : Inport  Port=5  LatchInput=off
  Cn_body : Inport  Port=6  LatchInput=off
  dcg2ac : Inport  Port=7  LatchInput=off
  Fcn4 : Fcn  Expr=u(4) - (u(2)*u(9) + u(3)*u(8))/Bref
  Fcn5 : Fcn  Expr=u(5) + (u(1)*u(9) - u(3)*u(7))/Cref
  Fcn6 : Fcn  Expr=u(6) + (u(2)*u(7) + u(1)*u(8))/Bref
  Mux1 : Mux  Inputs=7
  Cx_body : Outport
  Cy_body : Outport  Port=2
  Cz_body : Outport  Port=3
  CRcg : Outport  Port=4
  CMcg : Outport  Port=5
  CNcg : Outport  Port=6
  wires:
  Mux1/1 -> Fcn6/1, Fcn5/1, Fcn4/1
  dcg2ac/1 -> Mux1/7
  Cm_body/1 -> Mux1/5
  Cy/1 -> Cy_body/1, Mux1/2
  Fcn4/1 -> CRcg/1
  Fcn5/1 -> CMcg/1
  Fcn6/1 -> CNcg/1
  Cz/1 -> Cz_body/1, Mux1/3
  Cr_body/1 -> Mux1/4
  Cn_body/1 -> Mux1/6
  Cx/1 -> Cx_body/1, Mux1/1

== system AeroLib/Aircraft/Generic_Aircraft ==
  note: Generic Aircraft Model
      |  --------------------------------
      |  OPAL-RT Technologies
  Inputs : Inport  Port=1  LatchInput=off
  Aerodynamics_Generic : AeroLib/Aerodynamics/Aerodynamics_Generic
  AtmosphericData_FAA_gust : AeroLib/AtmosphericData/AtmosphericData_FAA_gust
  Autopilot : AeroLib/Autopilot/Autopilot
  Equations_of_Motion : AeroLib/EquationsOfMotion/Equations_of_Motion
  Landing_Gear : AeroLib/GroundReactions/Landing_Gear
  Mass_Properties : AeroLib/MassProperties/Mass_Properties
  Navigation_Sensors : AeroLib/Sensors/Navigation_Sensors
  Simple_Controls : AeroLib/Controls/Simple_Controls
  Stateless_Filter_Reset : AeroLib/AMS_StatelessFilters/Stateless_Filter_Reset
  Twin_Jet_Engine_system : AeroLib/Propulsion/Twin_Jet_Engine_system
  Sen_IRU_Out : Outport
  Sen_GPS_Out : Outport  Port=2
  Sen_FSC_Out : Outport  Port=3
  AP_Out : Outport  Port=4
  Ctrl_Out : Outport  Port=5
  EQM_Out : Outport  Port=6
  Atmos_Out : Outport  Port=7
  Prop_Out : Outport  Port=8
  wires:
  Mass_Properties/1 -> Equations_of_Motion/4
  AtmosphericData_FAA_gust/1 -> Atmos_Out/1, Aerodynamics_Generic/2, Navigation_Sensors/2, Twin_Jet_Engine_system/1
  Equations_of_Motion/1 -> Aerodynamics_Generic/3, AtmosphericData_FAA_gust/1, Navigation_Sensors/1, EQM_Out/1, Landing_Gear/3
  Aerodynamics_Generic/1 -> Equations_of_Motion/2
  Simple_Controls/1 -> Ctrl_Out/1, Aerodynamics_Generic/1, Twin_Jet_Engine_system/2
  Landing_Gear/1 -> Equations_of_Motion/1
  Autopilot/1 -> AP_Out/1, Simple_Controls/1, Landing_Gear/1
  Inputs/1 -> Autopilot/2, Aerodynamics_Generic/4, Twin_Jet_Engine_system/3, AtmosphericData_FAA_gust/2, Simple_Controls/2, Landing_Gear/2
  Stateless_Filter_Reset/1 -> Autopilot/3, Simple_Controls/3, Equations_of_Motion/5, AtmosphericData_FAA_gust/3, Twin_Jet_Engine_system/4, Navigation_Sensors/3
  Navigation_Sensors/3 -> Autopilot/1, Sen_FSC_Out/1
  Navigation_Sensors/1 -> Sen_IRU_Out/1
  Navigation_Sensors/2 -> Sen_GPS_Out/1
  Twin_Jet_Engine_system/1 -> Mass_Properties/1, Autopilot/4, Equations_of_Motion/3, Prop_Out/1

== system AeroLib/Aircraft/Pioneer_Aircraft ==
  note: Pioneer UAV Model
      |  --------------------------------
      |  OPAL-RT Technologies
  Inputs : Inport  Port=1  LatchInput=off
  Aerodynamics_Pioneer : AeroLib/Aerodynamics/Aerodynamics_Pioneer
  AtmosphericData_FAA_gust : AeroLib/AtmosphericData/AtmosphericData_FAA_gust
  Autopilot : AeroLib/Autopilot/Autopilot
  Equations_of_Motion : AeroLib/EquationsOfMotion/Equations_of_Motion
  Landing_Gear : AeroLib/GroundReactions/Landing_Gear
  Mass_Properties : AeroLib/MassProperties/Mass_Properties
  Navigation_Sensors : AeroLib/Sensors/Navigation_Sensors
  Piston_Engine_Propeller_system : AeroLib/Propulsion/Piston_Engine_Propeller_system
  Simple_Controls : AeroLib/Controls/Simple_Controls
  Stateless_Filter_Reset : AeroLib/AMS_StatelessFilters/Stateless_Filter_Reset
  Sen_IRU_Out : Outport
  Sen_GPS_Out : Outport  Port=2
  Sen_FSC_Out : Outport  Port=3
  AP_Out : Outport  Port=4
  Ctrl_Out : Outport  Port=5
  EQM_Out : Outport  Port=6
  Atmos_Out : Outport  Port=7
  Prop_Out : Outport  Port=8
  wires:
  Mass_Properties/1 -> Equations_of_Motion/4
  Equations_of_Motion/1 -> EQM_Out/1, Aerodynamics_Pioneer/3, AtmosphericData_FAA_gust/1, Navigation_Sensors/1, Landing_Gear/3
  Landing_Gear/1 -> Equations_of_Motion/1
  Piston_Engine_Propeller_system/1 -> Prop_Out/1, Autopilot/4, Equations_of_Motion/3, Mass_Properties/1
  Aerodynamics_Pioneer/1 -> Equations_of_Motion/2
  Autopilot/1 -> AP_Out/1, Simple_Controls/1, Landing_Gear/1
  AtmosphericData_FAA_gust/1 -> Atmos_Out/1, Navigation_Sensors/2, Aerodynamics_Pioneer/2, Piston_Engine_Propeller_system/1
  Simple_Controls/1 -> Ctrl_Out/1, Piston_Engine_Propeller_system/2, Aerodynamics_Pioneer/1
  Navigation_Sensors/3 -> Autopilot/1, Sen_FSC_Out/1
  Navigation_Sensors/2 -> Sen_GPS_Out/1
  Navigation_Sensors/1 -> Sen_IRU_Out/1
  Inputs/1 -> Piston_Engine_Propeller_system/3, Autopilot/2, Landing_Gear/2, Simple_Controls/2, AtmosphericData_FAA_gust/2
  Stateless_Filter_Reset/1 -> Piston_Engine_Propeller_system/4, Autopilot/3, Equations_of_Motion/5, AtmosphericData_FAA_gust/3, Simple_Controls/3, Navigation_Sensors/3

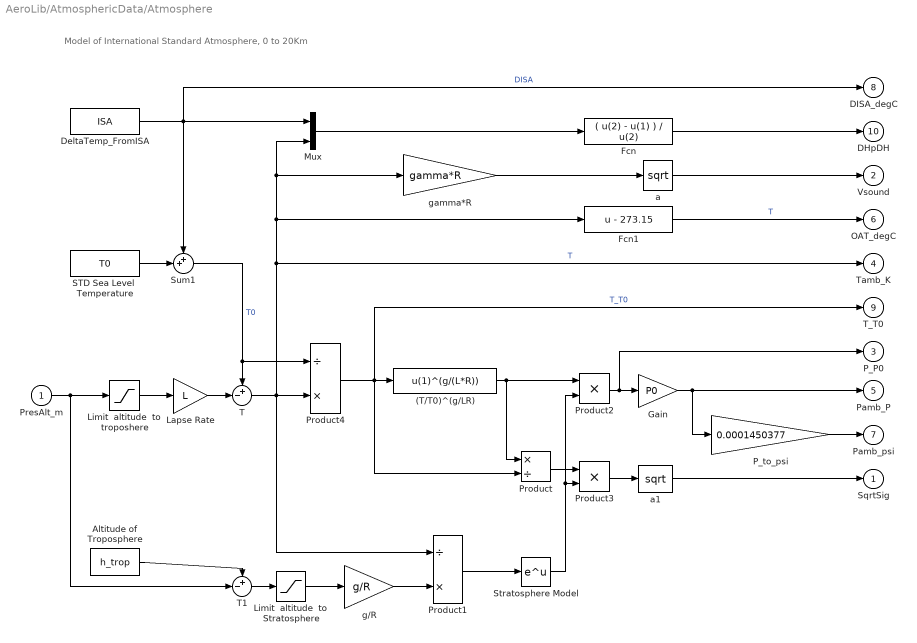
== system AeroLib/AtmosphericData/Atmosphere ==
  note: Model of International Standard Atmosphere, 0 to 20Km
  PresAlt_m : Inport  Port=1  LatchInput=off
  (T/T0)^(g/LR) : Fcn  Expr=u(1)^(g/(L*R))
  Altitude of Troposphere : Constant  Value=h_trop
  DeltaTemp_FromISA : Constant  Value=ISA
  Fcn : Fcn  Expr=( u(2) - u(1) ) / u(2)
  Fcn1 : Fcn  Expr=u - 273.15
  Gain : Gain  Gain=P0  SaturateOnIntegerOverflow=on
  Lapse Rate : Gain  Gain=L  SaturateOnIntegerOverflow=on
  Limit  altitude  to Stratosphere : Saturate  UpperLimit=0  LowerLimit=h_trop-20000
  Limit  altitude  to troposhere : Saturate  UpperLimit=h_trop  LowerLimit=0
  Mux : Mux  Inputs=2
  P_to_psi : Gain  Gain=0.0001450377  SaturateOnIntegerOverflow=on
  Product : Product  Inputs=*/  SaturateOnIntegerOverflow=on  InputSameDT=on
  Product1 : Product  Inputs=/*  SaturateOnIntegerOverflow=on  InputSameDT=on
  Product2 : Product  SaturateOnIntegerOverflow=on  InputSameDT=on
  Product3 : Product  SaturateOnIntegerOverflow=on  InputSameDT=on
  Product4 : Product  Inputs=/*  SaturateOnIntegerOverflow=on  InputSameDT=on
  STD Sea Level  Temperature : Constant  Value=T0
  Stratosphere Model : Math  SaturateOnIntegerOverflow=on
  Sum1 : Sum  Inputs=++|  SaturateOnIntegerOverflow=on  InputSameDT=on
  T : Sum  Inputs=+-|  SaturateOnIntegerOverflow=on  InputSameDT=on
  T1 : Sum  Inputs=+-|  SaturateOnIntegerOverflow=on  InputSameDT=on
  a : Math  Operator=sqrt  SaturateOnIntegerOverflow=on
  a1 : Math  Operator=sqrt  SaturateOnIntegerOverflow=on
  g/R : Gain  Gain=g/R  SaturateOnIntegerOverflow=on
  gamma*R : Gain  Gain=gamma*R  SaturateOnIntegerOverflow=on
  SqrtSig : Outport  InitialOutput=0
  "Vsound " : Outport  Port=2  InitialOutput=0
  "P_P0 " : Outport  Port=3  InitialOutput=0
  Tamb_K : Outport  Port=4  InitialOutput=0
  Pamb_P : Outport  Port=5  InitialOutput=0
  OAT_degC : Outport  Port=6  InitialOutput=0
  Pamb_psi : Outport  Port=7  InitialOutput=0
  DISA_degC : Outport  Port=8  InitialOutput=0
  T_T0 : Outport  Port=9  InitialOutput=0
  DHpDH : Outport  Port=10  InitialOutput=0
  wires:
  Sum1/1 -> Product4/1, T/1  "T0"
  Fcn/1 -> DHpDH/1
  Mux/1 -> Fcn/1
  PresAlt_m/1 -> T1/2, Limit  altitude  to troposhere/1
  Limit  altitude  to troposhere/1 -> Lapse Rate/1
  T/1 -> Tamb_K/1, gamma*R/1, Mux/2, Fcn1/1, Product4/2, Product1/1  "T"
  Product4/1 -> (T/T0)^(g/LR)/1, Product/2, T_T0/1  "T_T0"
  a1/1 -> SqrtSig/1
  Product/1 -> Product3/1
  (T/T0)^(g/LR)/1 -> Product2/1, Product/1
  gamma*R/1 -> a/1
  a/1 -> "Vsound "/1
  Lapse Rate/1 -> T/2
  STD Sea Level  Temperature/1 -> Sum1/2
  Product2/1 -> "P_P0 "/1, Gain/1
  Product3/1 -> a1/1
  Stratosphere Model/1 -> Product2/2, Product3/2
  g/R/1 -> Product1/2
  Product1/1 -> Stratosphere Model/1
  T1/1 -> Limit  altitude  to Stratosphere/1
  Limit  altitude  to Stratosphere/1 -> g/R/1
  Gain/1 -> Pamb_P/1, P_to_psi/1
  Fcn1/1 -> OAT_degC/1  "T"
  Altitude of Troposphere/1 -> T1/1
  DeltaTemp_FromISA/1 -> Sum1/1, Mux/1, DISA_degC/1  "DISA"
  P_to_psi/1 -> Pamb_psi/1

== system AeroLib/AtmosphericData/AtmosphericData_FAA_gust ==
  From_EQM : Inport  Port=1  LatchInput=off
  From_Inputs : Inport  Port=2  LatchInput=off
  From_Reset : Inport  Port=3  LatchInput=off
  Airspeeds : Subsystem
  Atmosphere : AeroLib/AtmosphericData/Atmosphere  ISA=Flight_delta_isa  g=9.806  gamma=1.4  R=287.0529  L=0.0065  h_trop=11000  P0=101325.0  T0=288.15
  Bus Creator : BusCreator  DialogController=Simulink.DDGSource_Bus  Inputs=20
  Bus Selector1 : BusSelector  DialogController=Simulink.DDGSource_Bus  OutputSignals=Vb,DCM,VD_mps
  Constant : Constant  Value=Flight_TurbON
  FAA_Std_Gust : AeroLib/AtmosphericData/FAA_Std_Gust
  Memory : Memory  X0=[0 0 0]
  Pressure_Altitude : Subsystem
  Terminator{,1..4} (5 alike) : Terminator
  Atmos_Out : Outport
  wires:
  Constant/1 -> FAA_Std_Gust/Enable
  Memory/1 -> Airspeeds/1(Wind)
  Bus Creator/1 -> Atmos_Out/1
  Pressure_Altitude/2(Hdot_mps) -> Bus Creator/19  "Hdot_mps"
  Atmosphere/6 -> Bus Creator/14  "OAT_degC"
  Atmosphere/5 -> Bus Creator/13  "Pamb_P"
  Pressure_Altitude/1(Pres_Alt_ft) -> Bus Creator/18  "PresAlt_ft"
  Airspeeds/4(TAS_kt) -> Bus Creator/4, FAA_Std_Gust/1  "TAS_kt"
  Airspeeds/5(Alpha) -> Bus Creator/5  "Alpha"
  Airspeeds/6(AlphaDot) -> Bus Creator/6  "AlphaDot"
  Airspeeds/7(Beta) -> Bus Creator/7  "Beta"
  Airspeeds/8(DynPres_Nm) -> Bus Creator/8  "DynPres_P"
  Airspeeds/9(DynPres_Kgf) -> Bus Creator/9  "DynPres_Kpm2"
  Atmosphere/1 -> Airspeeds/4(SqrtSig)
  Atmosphere/2 -> Airspeeds/5(Vsound)
  Atmosphere/10 -> Pressure_Altitude/1(DHpDH)
  Pressure_Altitude/3(Pres_Alt_m) -> Bus Creator/20, Atmosphere/1  "PresAlt_m"
  Airspeeds/1(KIAS_kt) -> Bus Creator/1  "KIAS"
  Airspeeds/2(Mach) -> Bus Creator/2  "Mach"
  Airspeeds/3(TAS_ms) -> Bus Creator/3  "TAS"
  From_EQM/1 -> Bus Selector1/1, FAA_Std_Gust/3
  Bus Selector1/1 -> Airspeeds/2(Vb)  "<Vb>"
  Bus Selector1/2 -> Airspeeds/3(DCM)  "<DCM>"
  Bus Selector1/3 -> Pressure_Altitude/2(VelI)  "<VD_mps>"
  Atmosphere/9 -> Bus Creator/17  "T_T0"
  Atmosphere/8 -> Bus Creator/16  "DISA_C"
  Atmosphere/4 -> Bus Creator/12  "Tamb_K"
  Atmosphere/7 -> Bus Creator/15  "Pamb_psi"
  Atmosphere/3 -> Bus Creator/11, Airspeeds/6(P_P0)  "P_P0"
  Airspeeds/10(BetaVt) -> Bus Creator/10  "BetaVT"
  From_Inputs/1 -> FAA_Std_Gust/2
  FAA_Std_Gust/1 -> Terminator4/1
  FAA_Std_Gust/2 -> Terminator3/1
  FAA_Std_Gust/3 -> Terminator2/1
  FAA_Std_Gust/4 -> Terminator/1
  FAA_Std_Gust/5 -> Terminator1/1
  FAA_Std_Gust/6 -> Memory/1
  From_Reset/1 -> FAA_Std_Gust/4

== system AeroLib/AtmosphericData/FAA_Std_Gust ==
  note: Flight_TurbON = 0 ==> No Turbulence
      |
      | Flight_TurbON = 0.2 ==> Light Turbulence
      |
      | Fligh_TurbON = 0.5 ==> Mild turbulence
      |
      | Flight_TurbON = 1 ==> Full Turbulence Model
  TAS_kt : Inport  Port=1  LatchInput=off
  From_Inputs : Inport  Port=2  LatchInput=off
  From_EQM : Inport  Port=3  LatchInput=off
  From_Reset : Inport  Port=4  LatchInput=off
  Enable : EnablePort
  Bus Selector1 : BusSelector  DialogController=Simulink.DDGSource_Bus  OutputSignals=Hagl_ft
  Inputs_to_WindXYZ : Subsystem
  MeanWind_Height_Profile : Subsystem
  Mux : Mux  Inputs=3
  Sum : Sum  Inputs=++|  SaturateOnIntegerOverflow=on  InputSameDT=on
  Sum1 : Sum  Inputs=++|  SaturateOnIntegerOverflow=on  InputSameDT=on
  Sum2 : Sum  Inputs=++|  SaturateOnIntegerOverflow=on  InputSameDT=on
  TASFilter : Subsystem
  Turbulence Parameters : Subsystem
  Turbulence U : Subsystem
  Turbulence V : Subsystem
  Turbulence W : Subsystem
  kt-->mps : Gain  Gain=Atm.kt_to_vel  SaturateOnIntegerOverflow=on
  mps-->kt : Gain  Gain=1.9438  SaturateOnIntegerOverflow=on
  WindX_kt : Outport
  WindY_kt : Outport  Port=2
  WindZ_kt : Outport  Port=3
  WindMag_kt : Outport  Port=4
  WindDir_deg : Outport  Port=5
  Wind_mps : Outport  Port=6
  wires:
  Sum1/1 -> WindY_kt/1, Mux/2
  From_EQM/1 -> Bus Selector1/1
  MeanWind_Height_Profile/5(WindDIr_deg) -> WindDir_deg/1
  MeanWind_Height_Profile/4(HorWind_kt) -> WindMag_kt/1
  kt-->mps/1 -> Wind_mps/1
  Mux/1 -> kt-->mps/1
  From_Inputs/1 -> Inputs_to_WindXYZ/1(From_Inputs)
  TAS_kt/1 -> TASFilter/1(TAS)
  TASFilter/1(TASFilt) -> Turbulence Parameters/3(TAS_kt)
  Turbulence Parameters/5(Noise_U) -> Turbulence U/1(Noise_U)  "Noise_U"
  MeanWind_Height_Profile/3(MeanWindZ_kt) -> Sum2/1
  MeanWind_Height_Profile/2(MeanWindY_kt) -> Sum1/1
  MeanWind_Height_Profile/1(MeanWindX_kt) -> Sum/1
  MeanWind_Height_Profile/6(MeanWind_kt) -> Turbulence Parameters/1(Wind_kt)
  Turbulence Parameters/4(TLW) -> Turbulence W/2(TLW)  "TLW"
  Turbulence Parameters/2(RMS_w) -> Turbulence W/3(RMS_w)  "RMS_w"
  Bus Selector1/1 -> Turbulence Parameters/2(Hagl_ft), MeanWind_Height_Profile/2(HAGL_ft)  "<Hagl_ft>"
  Turbulence V/1(V_turb) -> Sum1/2
  Turbulence W/1(Turb_W) -> Sum2/2
  Sum2/1 -> WindZ_kt/1, Mux/3
  Turbulence U/1(U_turb) -> Sum/2
  Sum/1 -> WindX_kt/1, Mux/1
  Turbulence Parameters/1(RMS_h) -> Turbulence V/3(RMS_H), Turbulence U/3(RMS_h)  "RMS_H"
  Turbulence Parameters/3(TLH) -> Turbulence U/2(TLH), Turbulence V/2(TLH)  "TLH"
  Turbulence Parameters/7(Noise_W) -> Turbulence W/1(Noise_w)  "Noise_W"
  Turbulence Parameters/6(Noise_V) -> Turbulence V/1(Noise_V)  "Noise_V"
  Inputs_to_WindXYZ/1(Wind_mps) -> mps-->kt/1
  From_Reset/1 -> Turbulence U/4(From_Reset), Turbulence V/4(From_Reset), Turbulence W/4(From_Reset)
  mps-->kt/1 -> MeanWind_Height_Profile/1(Wind_kt)
